simulink model "DSR_delay_beta_test"  (R2021a)
settings: Solver=VariableStepAuto  StartTime=0.0  StopTime=10  RelTol=1e-3
values from neighbouring files (symbols this model uses):
  a = 0    [gainMaxDef.m]    (also in plot2.m = 2; simulink_test.m = 5)
  alpha = 1.195    [gainMaxDef.m]    (also in plot2.m = 1.9; simulink_test.m = 1.192)
  betac = 2    [plot2.m]    (also in simulink_test.m = 10)
  c1 = 1    [simulink_test.m]
  delay = 0.5    [plot2.m]    (also in simulink_test.m = 0.015)
  delay_a = 0.150    (= 0.15)    [plot2.m]    (also in simulink_test.m = 0.01)
  gnet = 40    [plot2.m]    (also in simulink_test.m = gnetset(k))
  omega = omegalist(l)    [gainMaxDef.m]    (also in plot2.m = 300; simulink_test.m = 0.8)
  omegader = 80    [simulink_test.m]
undefined symbols (not defined in the file or in its folder): betacd
libraries: cstblocks x37, simulink x4
(part 1 of 3)
settings Model: Creator=shiva  LastModifiedBy=shiva

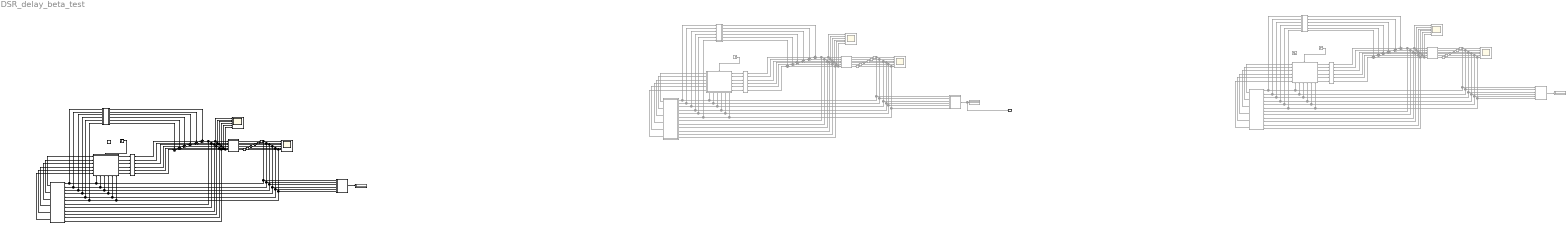
== system DSR_delay_beta_test ==
  note: DSR With CDOB
  note: DSR With CDOB
  note: DSR With CDOB
  CDOB_Subsys1 : Subsystem  Commented=on
  CDOB_Subsys2 : Subsystem  Commented=on
  CDOB_Subsys4 : Subsystem
  DSR_Input1 : Subsystem  Commented=on
      settings: PortSchema="{\"entries\":[{\"content\":{\"sides\":[{\"content\":{\"connectorIds\":[\"In1\",\"In2\",\"In3\",\"In4\",\"In5\",\"In6\"]},\"type\":\"ConnectorPlacement.EquallySpacedRectSide\",\"uuid\":\"7b8a38d4-2828-429e-a347-8750a0874c90\"},{\"content\":{\"connectorIds\":[\"Out1\",\"Out2\",\"Out3\",\"Out4\",\"Out5\",\"Out6\"],\"side\":\"RIGHT\"},\"type\":\"ConnectorPlacement.EquallySpacedRectSide\",\"uuid\":\"f1dcdaa7-0a93-43e2-be3b-ce942cee3b23\"},{\"content\":{\"connectorIds\":[\"In7\"],\"side\":\"TOP\"},\"type\":\"ConnectorPlacement.EquallySpacedRectSide\",\"uuid\":\"691a82b2-07cc-468b-b9a0-c0927a09fa47\"},{\"content\":{\"connectorIds\":[\"In8\",\"In9\",\"In10\",\"In11\",\"In12\",\"In13\"],\"side\":\"BOTTOM\"},\"type\":\"ConnectorPlacement.EquallySpacedRectSide\",\"uuid\":\"87ba8582-7e13-41cf-953e-972bab5f6463\"}]},\"type\":\"ConnectorPlacement.EquallySpacedConnector\",\"uuid\":\"6089c568-97aa-4e95-8448-5d1116d5973e\"}],\"packageUris\":[\"http://schema.mathworks.com/mf0/Connector/R2020b\"],\"version\":\"1.0\"}"
  DSR_Input2 : Subsystem  Commented=on
      settings: PortSchema="{\"entries\":[{\"content\":{\"sides\":[{\"content\":{\"connectorIds\":[\"In1\",\"In2\",\"In3\",\"In4\",\"In5\",\"In6\"]},\"type\":\"ConnectorPlacement.EquallySpacedRectSide\",\"uuid\":\"7b8a38d4-2828-429e-a347-8750a0874c90\"},{\"content\":{\"connectorIds\":[\"Out1\",\"Out2\",\"Out3\",\"Out4\",\"Out5\",\"Out6\"],\"side\":\"RIGHT\"},\"type\":\"ConnectorPlacement.EquallySpacedRectSide\",\"uuid\":\"f1dcdaa7-0a93-43e2-be3b-ce942cee3b23\"},{\"content\":{\"connectorIds\":[\"In7\"],\"side\":\"TOP\"},\"type\":\"ConnectorPlacement.EquallySpacedRectSide\",\"uuid\":\"691a82b2-07cc-468b-b9a0-c0927a09fa47\"},{\"content\":{\"connectorIds\":[\"In8\",\"In9\",\"In10\",\"In11\",\"In12\",\"In13\"],\"side\":\"BOTTOM\"},\"type\":\"ConnectorPlacement.EquallySpacedRectSide\",\"uuid\":\"87ba8582-7e13-41cf-953e-972bab5f6463\"}]},\"type\":\"ConnectorPlacement.EquallySpacedConnector\",\"uuid\":\"6089c568-97aa-4e95-8448-5d1116d5973e\"}],\"packageUris\":[\"http://schema.mathworks.com/mf0/Connector/R2020b\"],\"version\":\"1.0\"}"
  DSR_Input3 : Subsystem
      settings: PortSchema="{\"entries\":[{\"content\":{\"sides\":[{\"content\":{\"connectorIds\":[\"In1\",\"In2\",\"In3\",\"In4\",\"In5\",\"In6\"]},\"type\":\"ConnectorPlacement.EquallySpacedRectSide\",\"uuid\":\"7b8a38d4-2828-429e-a347-8750a0874c90\"},{\"content\":{\"connectorIds\":[\"Out1\",\"Out2\",\"Out3\",\"Out4\",\"Out5\",\"Out6\"],\"side\":\"RIGHT\"},\"type\":\"ConnectorPlacement.EquallySpacedRectSide\",\"uuid\":\"f1dcdaa7-0a93-43e2-be3b-ce942cee3b23\"},{\"content\":{\"connectorIds\":[\"In7\"],\"side\":\"TOP\"},\"type\":\"ConnectorPlacement.EquallySpacedRectSide\",\"uuid\":\"691a82b2-07cc-468b-b9a0-c0927a09fa47\"},{\"content\":{\"connectorIds\":[\"In8\",\"In9\",\"In10\",\"In11\",\"In12\",\"In13\"],\"side\":\"BOTTOM\"},\"type\":\"ConnectorPlacement.EquallySpacedRectSide\",\"uuid\":\"87ba8582-7e13-41cf-953e-972bab5f6463\"}]},\"type\":\"ConnectorPlacement.EquallySpacedConnector\",\"uuid\":\"6089c568-97aa-4e95-8448-5d1116d5973e\"}],\"packageUris\":[\"http://schema.mathworks.com/mf0/Connector/R2020b\"],\"version\":\"1.0\"}"
  Display1 : Display  Commented=on
  Display2 : Display
  Display3 : Display  Commented=on
  Max Deflection1 : Subsystem  Commented=on
  Max Deflection2 : Subsystem  Commented=on
  Max Deflection3 : Subsystem
  Ramp : simulink/Sources/Ramp  slope=1  start=0  InitialOutput=0
  Scope{1..4} (4 alike) : Scope  Commented=on  NumInputPorts=6
  Scope5 : Scope  NumInputPorts=6
  Scope6 : Scope  NumInputPorts=6
  Sine Wave1 : Sin  Commented=on  SampleTime=0
  StateDerivative1 : Subsystem  Commented=on
  StateDerivative2 : Subsystem  Commented=on
  StateDerivative3 : Subsystem
  Step1 : Step  Commented=on  Time=0  SampleTime=0
  Step2 : Step  Commented=on  Time=0  SampleTime=0
  Step3 : Step  Time=0  SampleTime=0
  Subsystem1 : Subsystem  Commented=on
  Subsystem2 : Subsystem
  Subsystem3 : Subsystem  Commented=on
  Sum{1..12} (12 alike) : Sum  Commented=on  Inputs=++|
  Sum{13..18} (6 alike) : Sum  Inputs=++|
  Transport Delay{1..12} (12 alike) : TransportDelay  Commented=on  DelayTime=delay_a
  Transport Delay{13..18} (6 alike) : TransportDelay  DelayTime=delay_a
  gain 1/a1 : Subsystem  Commented=on
  gain 1/a2 : Subsystem  Commented=on
  gain 1/a3 : Subsystem
  Output : Outport
  wires:
  Max Deflection1/1(y) -> Output/1, Display3/1
  Transport Delay3/1 -> StateDerivative1/2(Input1), CDOB_Subsys2/2(XRes1), DSR_Input1/9(s2), Max Deflection1/2(In2), Scope1/2
  Sum2/1 -> CDOB_Subsys2/8(Acc.1), Subsystem3/2(In2), Scope2/2
  DSR_Input1/1(Out1) -> gain 1/a1/1(In1)
  gain 1/a1/5(Out5) -> Sum5/2
  CDOB_Subsys2/4(FeedBack3) -> DSR_Input1/4(fb4)
  DSR_Input1/2(Out2) -> gain 1/a1/2(In2)
  Subsystem3/5(O5) -> Transport Delay11/1
  Subsystem3/2(O2) -> Transport Delay3/1
  DSR_Input1/4(Out4) -> gain 1/a1/4(In4)
  CDOB_Subsys2/1(FeedBack) -> DSR_Input1/1(fb1)
  gain 1/a1/6(Out6) -> Sum6/2
  Subsystem3/6(O6) -> Transport Delay2/1
  Sum4/1 -> CDOB_Subsys2/10(Acc.3), Scope2/4, Subsystem3/4(In4)
  DSR_Input1/6(Out6) -> gain 1/a1/6(In6)
  Transport Delay11/1 -> StateDerivative1/5(Input4), CDOB_Subsys2/5(XRes4), DSR_Input1/12(s5), Max Deflection1/5(In5), Scope1/5
  gain 1/a1/1(Out1) -> Sum1/2
  gain 1/a1/3(Out3) -> Sum3/2
  Sum6/1 -> Scope2/6, Subsystem3/6(In6), CDOB_Subsys2/12(Acc.5)
  DSR_Input1/5(Out5) -> gain 1/a1/5(In5)
  Subsystem3/3(O3) -> Transport Delay4/1
  DSR_Input1/3(Out3) -> gain 1/a1/3(In3)
  Sum3/1 -> CDOB_Subsys2/9(Acc.2), Scope2/3, Subsystem3/3(In3)
  Subsystem3/4(O4) -> Transport Delay5/1
  Transport Delay1/1 -> Scope1/1, StateDerivative1/1(Input), CDOB_Subsys2/1(XRes), DSR_Input1/8(s1), Max Deflection1/1(In1)
  Sum1/1 -> CDOB_Subsys2/7(Acc.), Subsystem3/1(In1), Scope2/1
  CDOB_Subsys2/5(FeedBack4) -> DSR_Input1/5(fb5)
  CDOB_Subsys2/6(FeedBack5) -> DSR_Input1/6(fb6)
  gain 1/a1/4(Out4) -> Sum4/2
  Transport Delay2/1 -> Scope1/6, StateDerivative1/6(Input5), CDOB_Subsys2/6(XRes5), DSR_Input1/13(s6), Max Deflection1/6(In6)
  gain 1/a1/2(Out2) -> Sum2/2
  Subsystem3/1(O1) -> Transport Delay1/1
  Transport Delay5/1 -> StateDerivative1/4(Input3), CDOB_Subsys2/4(XRes3), DSR_Input1/11(s4), Max Deflection1/4(In4), Scope1/4
  Transport Delay4/1 -> StateDerivative1/3(Input2), CDOB_Subsys2/3(XRes2), DSR_Input1/10(s3), Max Deflection1/3(In3), Scope1/3
  CDOB_Subsys2/2(FeedBack1) -> DSR_Input1/2(fb2)
  CDOB_Subsys2/3(FeedBack2) -> DSR_Input1/3(fb3)
  Sum5/1 -> CDOB_Subsys2/11(Acc.4), Scope2/5, Subsystem3/5(In5)
  StateDerivative1/1(Out1) -> Sum1/1
  StateDerivative1/2(Out2) -> Sum2/1
  StateDerivative1/3(Out3) -> Sum3/1
  StateDerivative1/4(Out4) -> Sum4/1
  StateDerivative1/5(Out5) -> Sum5/1
  StateDerivative1/6(Out6) -> Sum6/1
  Step1/1 -> DSR_Input1/7(input)
  StateDerivative2/4(Out4) -> Sum10/1
  StateDerivative2/2(Out2) -> Sum8/1
  StateDerivative2/3(Out3) -> Sum9/1
  StateDerivative2/1(Out1) -> Sum7/1
  Step2/1 -> DSR_Input2/7(input)
  DSR_Input2/2(Out2) -> gain 1/a2/2(In2)
  Max Deflection2/1(y) -> Display1/1
  Transport Delay10/1 -> StateDerivative2/3(Input2), CDOB_Subsys1/3(XRes2), DSR_Input2/10(s3), Max Deflection2/3(In3), Scope3/3
  Transport Delay12/1 -> StateDerivative2/4(Input3), CDOB_Subsys1/4(XRes3), DSR_Input2/11(s4), Max Deflection2/4(In4), Scope3/4
  Sum11/1 -> CDOB_Subsys1/11(Acc.4), Scope4/5, Subsystem1/5(In5)
  CDOB_Subsys1/3(FeedBack2) -> DSR_Input2/3(fb3)
  CDOB_Subsys1/2(FeedBack1) -> DSR_Input2/2(fb2)
  gain 1/a2/4(Out4) -> Sum10/2
  CDOB_Subsys1/6(FeedBack5) -> DSR_Input2/6(fb6)
  Subsystem1/4(O4) -> Transport Delay12/1
  CDOB_Subsys1/5(FeedBack4) -> DSR_Input2/5(fb5)
  Sum9/1 -> CDOB_Subsys1/9(Acc.2), Scope4/3, Subsystem1/3(In3)
  DSR_Input2/3(Out3) -> gain 1/a2/3(In3)
  StateDerivative2/6(Out6) -> Sum12/1
  Sum12/1 -> Scope4/6, Subsystem1/6(In6), CDOB_Subsys1/12(Acc.5)
  DSR_Input2/5(Out5) -> gain 1/a2/5(In5)
  gain 1/a2/1(Out1) -> Sum7/2
  Transport Delay7/1 -> StateDerivative2/5(Input4), CDOB_Subsys1/5(XRes4), DSR_Input2/12(s5), Max Deflection2/5(In5), Scope3/5
  gain 1/a2/3(Out3) -> Sum9/2
  gain 1/a2/2(Out2) -> Sum8/2
  Subsystem1/2(O2) -> Transport Delay9/1
  Subsystem1/6(O6) -> Transport Delay8/1
  Subsystem1/3(O3) -> Transport Delay10/1
  gain 1/a2/6(Out6) -> Sum12/2
  Sum10/1 -> CDOB_Subsys1/10(Acc.3), Scope4/4, Subsystem1/4(In4)
  Sum7/1 -> CDOB_Subsys1/7(Acc.), Subsystem1/1(In1), Scope4/1
  CDOB_Subsys1/1(FeedBack) -> DSR_Input2/1(fb1)
  DSR_Input2/4(Out4) -> gain 1/a2/4(In4)
  Subsystem1/5(O5) -> Transport Delay7/1
  Sum8/1 -> CDOB_Subsys1/8(Acc.1), Subsystem1/2(In2), Scope4/2
  CDOB_Subsys1/4(FeedBack3) -> DSR_Input2/4(fb4)
  DSR_Input2/6(Out6) -> gain 1/a2/6(In6)
  Transport Delay6/1 -> Scope3/1, StateDerivative2/1(Input), CDOB_Subsys1/1(XRes), DSR_Input2/8(s1), Max Deflection2/1(In1)
  StateDerivative2/5(Out5) -> Sum11/1
  Transport Delay8/1 -> StateDerivative2/6(Input5), CDOB_Subsys1/6(XRes5), DSR_Input2/13(s6), Max Deflection2/6(In6), Scope3/6
  gain 1/a2/5(Out5) -> Sum11/2
  DSR_Input2/1(Out1) -> gain 1/a2/1(In1)
  Subsystem1/1(O1) -> Transport Delay6/1
  Transport Delay9/1 -> StateDerivative2/2(Input1), CDOB_Subsys1/2(XRes1), DSR_Input2/9(s2), Max Deflection2/2(In2), Scope3/2
  StateDerivative3/3(Out3) -> Sum15/1
  DSR_Input3/6(Out6) -> gain 1/a3/6(In6)
  Transport Delay18/1 -> CDOB_Subsys4/4(XRes3), StateDerivative3/4(Input3), DSR_Input3/11(s4), Max Deflection3/4(In4), Scope5/4
  Sum13/1 -> CDOB_Subsys4/7(Acc.), Subsystem2/1(In1), Scope6/1
  gain 1/a3/2(Out2) -> Sum14/2
  gain 1/a3/3(Out3) -> Sum15/2
  StateDerivative3/2(Out2) -> Sum14/1
  gain 1/a3/5(Out5) -> Sum17/2
  CDOB_Subsys4/3(FeedBack2) -> DSR_Input3/3(fb3)
  Transport Delay16/1 -> CDOB_Subsys4/2(XRes1), StateDerivative3/2(Input1), DSR_Input3/9(s2), Max Deflection3/2(In2), Scope5/2
  DSR_Input3/3(Out3) -> gain 1/a3/3(In3)
  DSR_Input3/1(Out1) -> gain 1/a3/1(In1)
  Transport Delay17/1 -> CDOB_Subsys4/3(XRes2), StateDerivative3/3(Input2), DSR_Input3/10(s3), Max Deflection3/3(In3), Scope5/3
  Transport Delay14/1 -> CDOB_Subsys4/5(XRes4), StateDerivative3/5(Input4), DSR_Input3/12(s5), Max Deflection3/5(In5), Scope5/5
  Subsystem2/1(O1) -> Transport Delay13/1
  Transport Delay13/1 -> Scope5/1, CDOB_Subsys4/1(XRes), StateDerivative3/1(Input), DSR_Input3/8(s1), Max Deflection3/1(In1)
  StateDerivative3/4(Out4) -> Sum16/1
  StateDerivative3/1(Out1) -> Sum13/1
  gain 1/a3/4(Out4) -> Sum16/2
  CDOB_Subsys4/5(FeedBack4) -> DSR_Input3/5(fb5)
  Transport Delay15/1 -> Scope5/6, CDOB_Subsys4/6(XRes5), StateDerivative3/6(Input5), DSR_Input3/13(s6), Max Deflection3/6(In6)
  CDOB_Subsys4/1(FeedBack) -> DSR_Input3/1(fb1)
  Subsystem2/4(O4) -> Transport Delay18/1
  Sum17/1 -> CDOB_Subsys4/11(Acc.4), Scope6/5, Subsystem2/5(In5)
  CDOB_Subsys4/6(FeedBack5) -> DSR_Input3/6(fb6)
  Sum15/1 -> CDOB_Subsys4/9(Acc.2), Scope6/3, Subsystem2/3(In3)
  DSR_Input3/4(Out4) -> gain 1/a3/4(In4)
  Subsystem2/3(O3) -> Transport Delay17/1
  Subsystem2/2(O2) -> Transport Delay16/1
  Sum18/1 -> CDOB_Subsys4/12(Acc.5), Scope6/6, Subsystem2/6(In6)
  CDOB_Subsys4/4(FeedBack3) -> DSR_Input3/4(fb4)
  DSR_Input3/2(Out2) -> gain 1/a3/2(In2)
  Subsystem2/6(O6) -> Transport Delay15/1
  gain 1/a3/1(Out1) -> Sum13/2
  Sum16/1 -> CDOB_Subsys4/10(Acc.3), Scope6/4, Subsystem2/4(In4)
  gain 1/a3/6(Out6) -> Sum18/2
  DSR_Input3/5(Out5) -> gain 1/a3/5(In5)
  Max Deflection3/1(y) -> Display2/1
  StateDerivative3/5(Out5) -> Sum17/1
  StateDerivative3/6(Out6) -> Sum18/1
  Subsystem2/5(O5) -> Transport Delay14/1
  Sum14/1 -> CDOB_Subsys4/8(Acc.1), Subsystem2/2(In2), Scope6/2
  CDOB_Subsys4/2(FeedBack1) -> DSR_Input3/2(fb2)
  Step3/1 -> DSR_Input3/7(input)

== system DSR_delay_beta_test/CDOB_Subsys1 ==
  XRes : Inport
  XRes1 : Inport  Port=2
  XRes2 : Inport  Port=3
  XRes3 : Inport  Port=4
  XRes4 : Inport  Port=5
  XRes5 : Inport  Port=6
  Acc. : Inport  Port=7
  Acc.1 : Inport  Port=8
  Acc.2 : Inport  Port=9
  Acc.3 : Inport  Port=10
  Acc.4 : Inport  Port=11
  Acc.5 : Inport  Port=12
  ND : Subsystem
  ND1 : Subsystem
  ND2 : Subsystem
  ND3 : Subsystem
  ND4 : Subsystem
  ND5 : Subsystem
  FeedBack : Outport
  FeedBack1 : Outport  Port=2
  FeedBack2 : Outport  Port=3
  FeedBack3 : Outport  Port=4
  FeedBack4 : Outport  Port=5
  FeedBack5 : Outport  Port=6
  wires:
  Acc./1 -> ND/2(Acc.)
  XRes/1 -> ND/1(XRes)
  Acc.4/1 -> ND4/2(Acc.)
  Acc.3/1 -> ND3/2(Acc.)
  XRes1/1 -> ND1/1(XRes)
  XRes2/1 -> ND2/1(XRes)
  XRes4/1 -> ND4/1(XRes)
  XRes5/1 -> ND5/1(XRes)
  Acc.2/1 -> ND2/2(Acc.)
  ND5/1(FeedBack) -> FeedBack5/1
  ND1/1(FeedBack) -> FeedBack1/1
  ND2/1(FeedBack) -> FeedBack2/1
  Acc.5/1 -> ND5/2(Acc.)
  ND4/1(FeedBack) -> FeedBack4/1
  ND/1(FeedBack) -> FeedBack/1
  ND3/1(FeedBack) -> FeedBack3/1
  XRes3/1 -> ND3/1(XRes)
  Acc.1/1 -> ND1/2(Acc.)

== system DSR_delay_beta_test/CDOB_Subsys2 ==
  XRes : Inport
  XRes1 : Inport  Port=2
  XRes2 : Inport  Port=3
  XRes3 : Inport  Port=4
  XRes4 : Inport  Port=5
  XRes5 : Inport  Port=6
  Acc. : Inport  Port=7
  Acc.1 : Inport  Port=8
  Acc.2 : Inport  Port=9
  Acc.3 : Inport  Port=10
  Acc.4 : Inport  Port=11
  Acc.5 : Inport  Port=12
  ND : Subsystem
  ND1 : Subsystem
  ND2 : Subsystem
  ND3 : Subsystem
  ND4 : Subsystem
  ND5 : Subsystem
  FeedBack : Outport
  FeedBack1 : Outport  Port=2
  FeedBack2 : Outport  Port=3
  FeedBack3 : Outport  Port=4
  FeedBack4 : Outport  Port=5
  FeedBack5 : Outport  Port=6
  wires:
  Acc./1 -> ND/2(Acc.)
  XRes/1 -> ND/1(XRes)
  Acc.4/1 -> ND4/2(Acc.)
  Acc.3/1 -> ND3/2(Acc.)
  XRes1/1 -> ND1/1(XRes)
  XRes2/1 -> ND2/1(XRes)
  XRes4/1 -> ND4/1(XRes)
  XRes5/1 -> ND5/1(XRes)
  Acc.2/1 -> ND2/2(Acc.)
  ND5/1(FeedBack) -> FeedBack5/1
  ND1/1(FeedBack) -> FeedBack1/1
  ND2/1(FeedBack) -> FeedBack2/1
  Acc.5/1 -> ND5/2(Acc.)
  ND4/1(FeedBack) -> FeedBack4/1
  ND/1(FeedBack) -> FeedBack/1
  ND3/1(FeedBack) -> FeedBack3/1
  XRes3/1 -> ND3/1(XRes)
  Acc.1/1 -> ND1/2(Acc.)

== system DSR_delay_beta_test/CDOB_Subsys4 ==
  XRes : Inport
  XRes1 : Inport  Port=2
  XRes2 : Inport  Port=3
  XRes3 : Inport  Port=4
  XRes4 : Inport  Port=5
  XRes5 : Inport  Port=6
  Acc. : Inport  Port=7
  Acc.1 : Inport  Port=8
  Acc.2 : Inport  Port=9
  Acc.3 : Inport  Port=10
  Acc.4 : Inport  Port=11
  Acc.5 : Inport  Port=12
  ND : Subsystem
  ND1 : Subsystem
  ND2 : Subsystem
  ND3 : Subsystem
  ND4 : Subsystem
  ND5 : Subsystem
  FeedBack : Outport
  FeedBack1 : Outport  Port=2
  FeedBack2 : Outport  Port=3
  FeedBack3 : Outport  Port=4
  FeedBack4 : Outport  Port=5
  FeedBack5 : Outport  Port=6
  wires:
  Acc./1 -> ND/2(Acc.)
  XRes/1 -> ND/1(XRes)
  Acc.4/1 -> ND4/2(Acc.)
  Acc.3/1 -> ND3/2(Acc.)
  XRes1/1 -> ND1/1(XRes)
  XRes2/1 -> ND2/1(XRes)
  XRes4/1 -> ND4/1(XRes)
  XRes5/1 -> ND5/1(XRes)
  Acc.2/1 -> ND2/2(Acc.)
  ND5/1(FeedBack) -> FeedBack5/1
  ND1/1(FeedBack) -> FeedBack1/1
  ND2/1(FeedBack) -> FeedBack2/1
  Acc.5/1 -> ND5/2(Acc.)
  ND4/1(FeedBack) -> FeedBack4/1
  ND/1(FeedBack) -> FeedBack/1
  ND3/1(FeedBack) -> FeedBack3/1
  XRes3/1 -> ND3/1(XRes)
  Acc.1/1 -> ND1/2(Acc.)

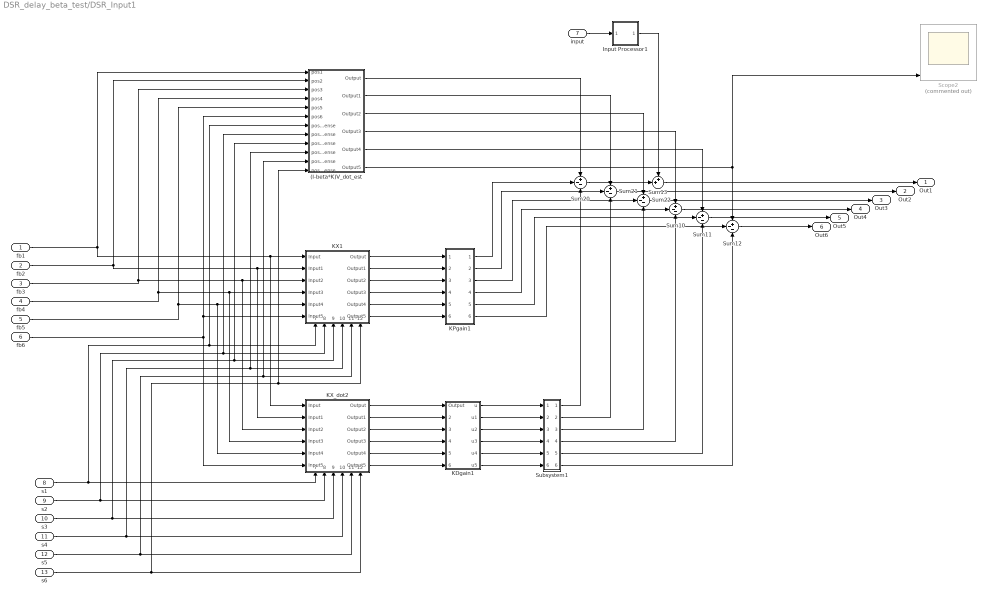
== system DSR_delay_beta_test/DSR_Input1 ==
  fb1 : Inport
  fb2 : Inport  Port=2
  fb3 : Inport  Port=3
  fb4 : Inport  Port=4
  fb5 : Inport  Port=5
  fb6 : Inport  Port=6
  input : Inport  Port=7
  s1 : Inport  Port=8
  s2 : Inport  Port=9
  s3 : Inport  Port=10
  s4 : Inport  Port=11
  s5 : Inport  Port=12
  s6 : Inport  Port=13
  (I-beta*K)V_dot_est : Subsystem
  Input Processor1 : Subsystem
  KDgain1 : Subsystem
  KPgain1 : Subsystem
  KX1 : Subsystem
      settings: PortSchema="{\"entries\":[{\"content\":{\"sides\":[{\"content\":{\"connectorIds\":[\"In1\",\"In2\",\"In3\",\"In4\",\"In5\",\"In6\"]},\"type\":\"ConnectorPlacement.EquallySpacedRectSide\",\"uuid\":\"24ff0189-2e26-4de2-9c90-2043606e3d63\"},{\"content\":{\"connectorIds\":[\"Out1\",\"Out2\",\"Out3\",\"Out4\",\"Out5\",\"Out6\"],\"side\":\"RIGHT\"},\"type\":\"ConnectorPlacement.EquallySpacedRectSide\",\"uuid\":\"7efe01dd-8101-429e-adc6-a10b45356e48\"},{\"content\":{\"connectorIds\":[],\"side\":\"TOP\"},\"type\":\"ConnectorPlacement.EquallySpacedRectSide\",\"uuid\":\"5c1fc1f4-b8b0-4afd-80fe-11f4d157d0fc\"},{\"content\":{\"connectorIds\":[\"In7\",\"In8\",\"In9\",\"In10\",\"In11\",\"In12\"],\"side\":\"BOTTOM\"},\"type\":\"ConnectorPlacement.EquallySpacedRectSide\",\"uuid\":\"e52c51d8-b236-4cc8-9958-a8d91e3741c4\"}]},\"type\":\"ConnectorPlacement.EquallySpacedConnector\",\"uuid\":\"3e3502e3-b8a3-4e9d-9b78-ab08dd870d4b\"}],\"packageUris\":[\"http://schema.mathworks.com/mf0/Connector/R2020b\"],\"version\":\"1.0\"}"
  KX_dot2 : Subsystem
      settings: PortSchema="{\"entries\":[{\"content\":{\"sides\":[{\"content\":{\"connectorIds\":[\"In1\",\"In2\",\"In3\",\"In4\",\"In5\",\"In6\"]},\"type\":\"ConnectorPlacement.EquallySpacedRectSide\",\"uuid\":\"24ff0189-2e26-4de2-9c90-2043606e3d63\"},{\"content\":{\"connectorIds\":[\"Out1\",\"Out2\",\"Out3\",\"Out4\",\"Out5\",\"Out6\"],\"side\":\"RIGHT\"},\"type\":\"ConnectorPlacement.EquallySpacedRectSide\",\"uuid\":\"7efe01dd-8101-429e-adc6-a10b45356e48\"},{\"content\":{\"connectorIds\":[],\"side\":\"TOP\"},\"type\":\"ConnectorPlacement.EquallySpacedRectSide\",\"uuid\":\"5c1fc1f4-b8b0-4afd-80fe-11f4d157d0fc\"},{\"content\":{\"connectorIds\":[\"In7\",\"In8\",\"In9\",\"In10\",\"In11\",\"In12\"],\"side\":\"BOTTOM\"},\"type\":\"ConnectorPlacement.EquallySpacedRectSide\",\"uuid\":\"bae418dc-ca78-4370-85bb-31cb43009c14\"}]},\"type\":\"ConnectorPlacement.EquallySpacedConnector\",\"uuid\":\"3e3502e3-b8a3-4e9d-9b78-ab08dd870d4b\"}],\"packageUris\":[\"http://schema.mathworks.com/mf0/Connector/R2020b\"],\"version\":\"1.0\"}"
  Scope2 : Scope  Commented=on  NumInputPorts=6
  Subsystem1 : Subsystem
  Sum{10..12,20..22} (6 alike) : Sum  Inputs=+--
  Sum13 : Sum  Inputs=++|
  Out1 : Outport
  Out2 : Outport  Port=2
  Out3 : Outport  Port=3
  Out4 : Outport  Port=4
  Out5 : Outport  Port=5
  Out6 : Outport  Port=6
  wires:
  KX_dot2/5(Output4) -> KDgain1/5(Output4)
  fb4/1 -> KX1/4(Input3), KX_dot2/4(Input3), (I-beta*K)V_dot_est/4(pos4)
  fb2/1 -> KX1/2(Input1), KX_dot2/2(Input1), (I-beta*K)V_dot_est/2(pos2)
  KDgain1/6(u5) -> Subsystem1/6(u5)
  fb3/1 -> KX1/3(Input2), KX_dot2/3(Input2), (I-beta*K)V_dot_est/3(pos3)
  KPgain1/4(Out4) -> Sum10/2
  Sum10/1 -> Out4/1
  KPgain1/2(Out2) -> Sum21/2
  KX1/6(Output5) -> KPgain1/6(Output5)
  KX1/2(Output1) -> KPgain1/2(Output1)
  KPgain1/6(Out6) -> Sum12/2
  KX1/4(Output3) -> KPgain1/4(Output3)
  KX1/3(Output2) -> KPgain1/3(Output2)
  s6/1 -> KX_dot2/12(sense6), (I-beta*K)V_dot_est/12(pos6sense), KX1/12(sense6)
  KDgain1/4(u3) -> Subsystem1/4(u3)
  fb5/1 -> KX1/5(Input4), KX_dot2/5(Input4), (I-beta*K)V_dot_est/5(pos5)
  Sum22/1 -> Out3/1
  Sum12/1 -> Out6/1
  KPgain1/3(Out3) -> Sum22/2
  KDgain1/5(u4) -> Subsystem1/5(u4)
  KDgain1/2(u1) -> Subsystem1/2(u1)
  s3/1 -> KX_dot2/9(sense3), (I-beta*K)V_dot_est/9(pos3sense), KX1/9(sense3)
  Sum20/1 -> Sum13/2
  KDgain1/3(u2) -> Subsystem1/3(u2)
  KX_dot2/4(Output3) -> KDgain1/4(Output3)
  fb1/1 -> KX1/1(Input), KX_dot2/1(Input), (I-beta*K)V_dot_est/1(pos1)
  (I-beta*K)V_dot_est/1(Output) -> Sum20/1
  KX_dot2/6(Output5) -> KDgain1/6(Output5)
  s1/1 -> KX_dot2/7(sense1), (I-beta*K)V_dot_est/7(pos1sense), KX1/7(sense1)
  s5/1 -> KX_dot2/11(sense5), (I-beta*K)V_dot_est/11(pos5sense), KX1/11(sense5)
  KX_dot2/2(Output1) -> KDgain1/2(Output1)
  Sum21/1 -> Out2/1
  KPgain1/5(Out5) -> Sum11/2
  fb6/1 -> KX1/6(Input5), (I-beta*K)V_dot_est/6(pos6), KX_dot2/6(Input5)
  (I-beta*K)V_dot_est/3(Output2) -> Sum22/1
  s4/1 -> KX_dot2/10(sense4), (I-beta*K)V_dot_est/10(pos4sense), KX1/10(sense4)
  KX1/5(Output4) -> KPgain1/5(Output4)
  KDgain1/1(u) -> Subsystem1/1(u)
  KX1/1(Output) -> KPgain1/1(Output)
  input/1 -> Input Processor1/1(Input)
  (I-beta*K)V_dot_est/2(Output1) -> Sum21/1
  KX_dot2/3(Output2) -> KDgain1/3(Output2)
  Sum11/1 -> Out5/1
  (I-beta*K)V_dot_est/4(Output3) -> Sum10/1
  KX_dot2/1(Output) -> KDgain1/1(Output)
  (I-beta*K)V_dot_est/5(Output4) -> Sum11/1
  (I-beta*K)V_dot_est/6(Output5) -> Scope2/6, Sum12/1
  KPgain1/1(Out1) -> Sum20/2
  s2/1 -> KX_dot2/8(sense2), (I-beta*K)V_dot_est/8(pos2sense), KX1/8(sense2)
  Sum13/1 -> Out1/1
  Input Processor1/1(Out1) -> Sum13/1
  Subsystem1/1(Out7) -> Sum20/3
  Subsystem1/2(Out8) -> Sum21/3
  Subsystem1/3(Out9) -> Sum22/3
  Subsystem1/4(Out10) -> Sum10/3
  Subsystem1/5(Out11) -> Sum11/3
  Subsystem1/6(Out12) -> Sum12/3

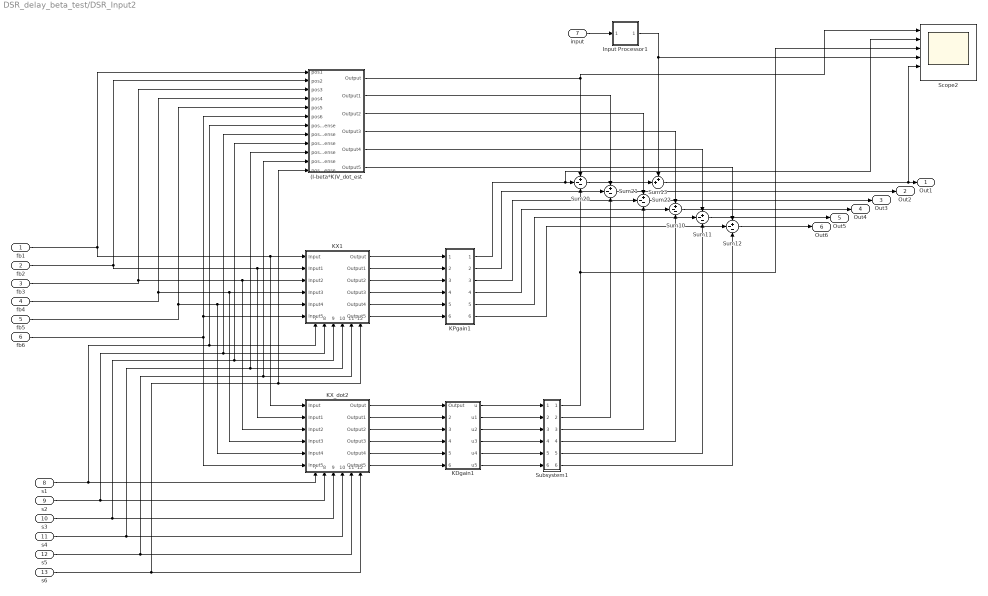
== system DSR_delay_beta_test/DSR_Input2 ==
  fb1 : Inport
  fb2 : Inport  Port=2
  fb3 : Inport  Port=3
  fb4 : Inport  Port=4
  fb5 : Inport  Port=5
  fb6 : Inport  Port=6
  input : Inport  Port=7
  s1 : Inport  Port=8
  s2 : Inport  Port=9
  s3 : Inport  Port=10
  s4 : Inport  Port=11
  s5 : Inport  Port=12
  s6 : Inport  Port=13
  (I-beta*K)V_dot_est : Subsystem
  Input Processor1 : Subsystem
  KDgain1 : Subsystem
  KPgain1 : Subsystem
  KX1 : Subsystem
      settings: PortSchema="{\"entries\":[{\"content\":{\"sides\":[{\"content\":{\"connectorIds\":[\"In1\",\"In2\",\"In3\",\"In4\",\"In5\",\"In6\"]},\"type\":\"ConnectorPlacement.EquallySpacedRectSide\",\"uuid\":\"24ff0189-2e26-4de2-9c90-2043606e3d63\"},{\"content\":{\"connectorIds\":[\"Out1\",\"Out2\",\"Out3\",\"Out4\",\"Out5\",\"Out6\"],\"side\":\"RIGHT\"},\"type\":\"ConnectorPlacement.EquallySpacedRectSide\",\"uuid\":\"7efe01dd-8101-429e-adc6-a10b45356e48\"},{\"content\":{\"connectorIds\":[],\"side\":\"TOP\"},\"type\":\"ConnectorPlacement.EquallySpacedRectSide\",\"uuid\":\"5c1fc1f4-b8b0-4afd-80fe-11f4d157d0fc\"},{\"content\":{\"connectorIds\":[\"In7\",\"In8\",\"In9\",\"In10\",\"In11\",\"In12\"],\"side\":\"BOTTOM\"},\"type\":\"ConnectorPlacement.EquallySpacedRectSide\",\"uuid\":\"e52c51d8-b236-4cc8-9958-a8d91e3741c4\"}]},\"type\":\"ConnectorPlacement.EquallySpacedConnector\",\"uuid\":\"3e3502e3-b8a3-4e9d-9b78-ab08dd870d4b\"}],\"packageUris\":[\"http://schema.mathworks.com/mf0/Connector/R2020b\"],\"version\":\"1.0\"}"
  KX_dot2 : Subsystem
      settings: PortSchema="{\"entries\":[{\"content\":{\"sides\":[{\"content\":{\"connectorIds\":[\"In1\",\"In2\",\"In3\",\"In4\",\"In5\",\"In6\"]},\"type\":\"ConnectorPlacement.EquallySpacedRectSide\",\"uuid\":\"24ff0189-2e26-4de2-9c90-2043606e3d63\"},{\"content\":{\"connectorIds\":[\"Out1\",\"Out2\",\"Out3\",\"Out4\",\"Out5\",\"Out6\"],\"side\":\"RIGHT\"},\"type\":\"ConnectorPlacement.EquallySpacedRectSide\",\"uuid\":\"7efe01dd-8101-429e-adc6-a10b45356e48\"},{\"content\":{\"connectorIds\":[],\"side\":\"TOP\"},\"type\":\"ConnectorPlacement.EquallySpacedRectSide\",\"uuid\":\"5c1fc1f4-b8b0-4afd-80fe-11f4d157d0fc\"},{\"content\":{\"connectorIds\":[\"In7\",\"In8\",\"In9\",\"In10\",\"In11\",\"In12\"],\"side\":\"BOTTOM\"},\"type\":\"ConnectorPlacement.EquallySpacedRectSide\",\"uuid\":\"bae418dc-ca78-4370-85bb-31cb43009c14\"}]},\"type\":\"ConnectorPlacement.EquallySpacedConnector\",\"uuid\":\"3e3502e3-b8a3-4e9d-9b78-ab08dd870d4b\"}],\"packageUris\":[\"http://schema.mathworks.com/mf0/Connector/R2020b\"],\"version\":\"1.0\"}"
  Scope2 : Scope  NumInputPorts=6
  Subsystem1 : Subsystem
  Sum{10..12,20..22} (6 alike) : Sum  Inputs=+--
  Sum13 : Sum  Inputs=++|
  Out1 : Outport
  Out2 : Outport  Port=2
  Out3 : Outport  Port=3
  Out4 : Outport  Port=4
  Out5 : Outport  Port=5
  Out6 : Outport  Port=6
  wires:
  KX_dot2/5(Output4) -> KDgain1/5(Output4)
  fb4/1 -> KX1/4(Input3), KX_dot2/4(Input3), (I-beta*K)V_dot_est/4(pos4)
  fb2/1 -> KX1/2(Input1), KX_dot2/2(Input1), (I-beta*K)V_dot_est/2(pos2)
  KDgain1/6(u5) -> Subsystem1/6(u5)
  fb3/1 -> KX1/3(Input2), KX_dot2/3(Input2), (I-beta*K)V_dot_est/3(pos3)
  KPgain1/4(Out4) -> Sum10/2
  Sum10/1 -> Out4/1
  KPgain1/2(Out2) -> Sum21/2
  KX1/6(Output5) -> KPgain1/6(Output5)
  KX1/2(Output1) -> KPgain1/2(Output1)
  KPgain1/6(Out6) -> Sum12/2
  KX1/4(Output3) -> KPgain1/4(Output3)
  KX1/3(Output2) -> KPgain1/3(Output2)
  s6/1 -> KX_dot2/12(sense6), (I-beta*K)V_dot_est/12(pos6sense), KX1/12(sense6)
  KDgain1/4(u3) -> Subsystem1/4(u3)
  fb5/1 -> KX1/5(Input4), KX_dot2/5(Input4), (I-beta*K)V_dot_est/5(pos5)
  Sum22/1 -> Out3/1
  Sum12/1 -> Out6/1
  KPgain1/3(Out3) -> Sum22/2
  KDgain1/5(u4) -> Subsystem1/5(u4)
  KDgain1/2(u1) -> Subsystem1/2(u1)
  s3/1 -> KX_dot2/9(sense3), (I-beta*K)V_dot_est/9(pos3sense), KX1/9(sense3)
  Sum20/1 -> Sum13/2
  KDgain1/3(u2) -> Subsystem1/3(u2)
  KX_dot2/4(Output3) -> KDgain1/4(Output3)
  fb1/1 -> KX1/1(Input), KX_dot2/1(Input), (I-beta*K)V_dot_est/1(pos1)
  (I-beta*K)V_dot_est/1(Output) -> Scope2/1, Sum20/1
  KX_dot2/6(Output5) -> KDgain1/6(Output5)
  s1/1 -> KX_dot2/7(sense1), (I-beta*K)V_dot_est/7(pos1sense), KX1/7(sense1)
  s5/1 -> KX_dot2/11(sense5), (I-beta*K)V_dot_est/11(pos5sense), KX1/11(sense5)
  KX_dot2/2(Output1) -> KDgain1/2(Output1)
  Sum21/1 -> Out2/1
  KPgain1/5(Out5) -> Sum11/2
  fb6/1 -> KX1/6(Input5), (I-beta*K)V_dot_est/6(pos6), KX_dot2/6(Input5)
  (I-beta*K)V_dot_est/3(Output2) -> Sum22/1
  s4/1 -> KX_dot2/10(sense4), (I-beta*K)V_dot_est/10(pos4sense), KX1/10(sense4)
  KX1/5(Output4) -> KPgain1/5(Output4)
  KDgain1/1(u) -> Subsystem1/1(u)
  KX1/1(Output) -> KPgain1/1(Output)
  input/1 -> Input Processor1/1(Input)
  (I-beta*K)V_dot_est/2(Output1) -> Sum21/1
  KX_dot2/3(Output2) -> KDgain1/3(Output2)
  Sum11/1 -> Out5/1
  (I-beta*K)V_dot_est/4(Output3) -> Sum10/1
  KX_dot2/1(Output) -> KDgain1/1(Output)
  (I-beta*K)V_dot_est/5(Output4) -> Sum11/1
  (I-beta*K)V_dot_est/6(Output5) -> Sum12/1
  KPgain1/1(Out1) -> Scope2/2, Sum20/2
  s2/1 -> KX_dot2/8(sense2), (I-beta*K)V_dot_est/8(pos2sense), KX1/8(sense2)
  Sum13/1 -> Scope2/5, Out1/1
  Input Processor1/1(Out1) -> Scope2/4, Sum13/1
  Subsystem1/1(Out7) -> Scope2/3, Sum20/3
  Subsystem1/2(Out8) -> Sum21/3
  Subsystem1/3(Out9) -> Sum22/3
  Subsystem1/4(Out10) -> Sum10/3
  Subsystem1/5(Out11) -> Sum11/3
  Subsystem1/6(Out12) -> Sum12/3

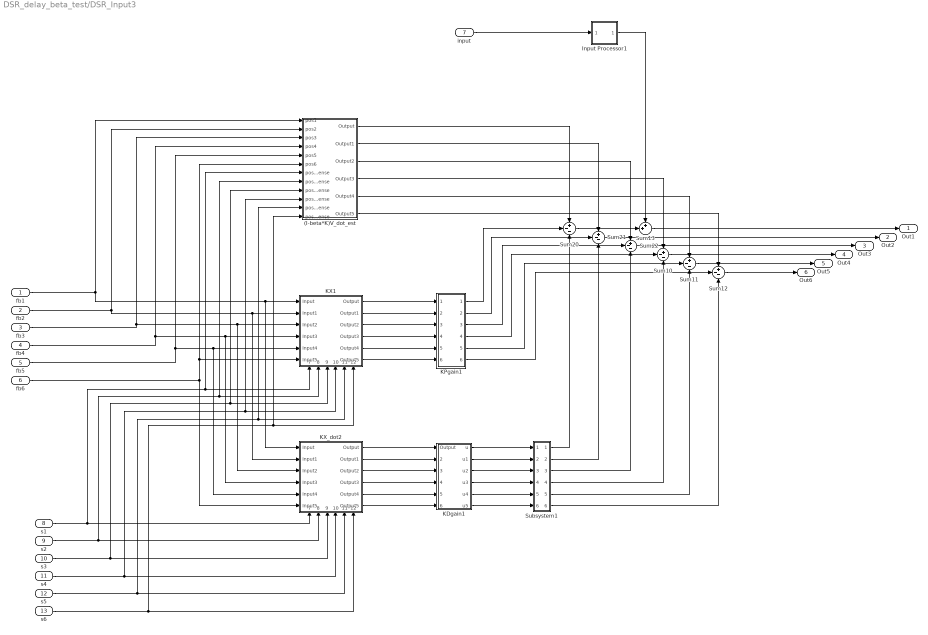
== system DSR_delay_beta_test/DSR_Input3 ==
  fb1 : Inport
  fb2 : Inport  Port=2
  fb3 : Inport  Port=3
  fb4 : Inport  Port=4
  fb5 : Inport  Port=5
  fb6 : Inport  Port=6
  input : Inport  Port=7
  s1 : Inport  Port=8
  s2 : Inport  Port=9
  s3 : Inport  Port=10
  s4 : Inport  Port=11
  s5 : Inport  Port=12
  s6 : Inport  Port=13
  (I-beta*K)V_dot_est : Subsystem
  Input Processor1 : Subsystem
  KDgain1 : Subsystem
  KPgain1 : Subsystem
  KX1 : Subsystem
      settings: PortSchema="{\"entries\":[{\"content\":{\"sides\":[{\"content\":{\"connectorIds\":[\"In1\",\"In2\",\"In3\",\"In4\",\"In5\",\"In6\"]},\"type\":\"ConnectorPlacement.EquallySpacedRectSide\",\"uuid\":\"24ff0189-2e26-4de2-9c90-2043606e3d63\"},{\"content\":{\"connectorIds\":[\"Out1\",\"Out2\",\"Out3\",\"Out4\",\"Out5\",\"Out6\"],\"side\":\"RIGHT\"},\"type\":\"ConnectorPlacement.EquallySpacedRectSide\",\"uuid\":\"7efe01dd-8101-429e-adc6-a10b45356e48\"},{\"content\":{\"connectorIds\":[],\"side\":\"TOP\"},\"type\":\"ConnectorPlacement.EquallySpacedRectSide\",\"uuid\":\"5c1fc1f4-b8b0-4afd-80fe-11f4d157d0fc\"},{\"content\":{\"connectorIds\":[\"In7\",\"In8\",\"In9\",\"In10\",\"In11\",\"In12\"],\"side\":\"BOTTOM\"},\"type\":\"ConnectorPlacement.EquallySpacedRectSide\",\"uuid\":\"e52c51d8-b236-4cc8-9958-a8d91e3741c4\"}]},\"type\":\"ConnectorPlacement.EquallySpacedConnector\",\"uuid\":\"3e3502e3-b8a3-4e9d-9b78-ab08dd870d4b\"}],\"packageUris\":[\"http://schema.mathworks.com/mf0/Connector/R2020b\"],\"version\":\"1.0\"}"
  KX_dot2 : Subsystem
      settings: PortSchema="{\"entries\":[{\"content\":{\"sides\":[{\"content\":{\"connectorIds\":[\"In1\",\"In2\",\"In3\",\"In4\",\"In5\",\"In6\"]},\"type\":\"ConnectorPlacement.EquallySpacedRectSide\",\"uuid\":\"24ff0189-2e26-4de2-9c90-2043606e3d63\"},{\"content\":{\"connectorIds\":[\"Out1\",\"Out2\",\"Out3\",\"Out4\",\"Out5\",\"Out6\"],\"side\":\"RIGHT\"},\"type\":\"ConnectorPlacement.EquallySpacedRectSide\",\"uuid\":\"7efe01dd-8101-429e-adc6-a10b45356e48\"},{\"content\":{\"connectorIds\":[],\"side\":\"TOP\"},\"type\":\"ConnectorPlacement.EquallySpacedRectSide\",\"uuid\":\"5c1fc1f4-b8b0-4afd-80fe-11f4d157d0fc\"},{\"content\":{\"connectorIds\":[\"In7\",\"In8\",\"In9\",\"In10\",\"In11\",\"In12\"],\"side\":\"BOTTOM\"},\"type\":\"ConnectorPlacement.EquallySpacedRectSide\",\"uuid\":\"bae418dc-ca78-4370-85bb-31cb43009c14\"}]},\"type\":\"ConnectorPlacement.EquallySpacedConnector\",\"uuid\":\"3e3502e3-b8a3-4e9d-9b78-ab08dd870d4b\"}],\"packageUris\":[\"http://schema.mathworks.com/mf0/Connector/R2020b\"],\"version\":\"1.0\"}"
  Subsystem1 : Subsystem
  Sum{10..12,20..22} (6 alike) : Sum  Inputs=+--
  Sum13 : Sum  Inputs=++|
  Out1 : Outport
  Out2 : Outport  Port=2
  Out3 : Outport  Port=3
  Out4 : Outport  Port=4
  Out5 : Outport  Port=5
  Out6 : Outport  Port=6
  wires:
  KX_dot2/5(Output4) -> KDgain1/5(Output4)
  fb4/1 -> KX1/4(Input3), KX_dot2/4(Input3), (I-beta*K)V_dot_est/4(pos4)
  fb2/1 -> KX1/2(Input1), KX_dot2/2(Input1), (I-beta*K)V_dot_est/2(pos2)
  KDgain1/6(u5) -> Subsystem1/6(u5)
  fb3/1 -> KX1/3(Input2), KX_dot2/3(Input2), (I-beta*K)V_dot_est/3(pos3)
  KPgain1/4(Out4) -> Sum10/2
  Sum10/1 -> Out4/1
  KPgain1/2(Out2) -> Sum21/2
  KX1/6(Output5) -> KPgain1/6(Output5)
  KX1/2(Output1) -> KPgain1/2(Output1)
  KPgain1/6(Out6) -> Sum12/2
  KX1/4(Output3) -> KPgain1/4(Output3)
  KX1/3(Output2) -> KPgain1/3(Output2)
  s6/1 -> KX_dot2/12(sense6), (I-beta*K)V_dot_est/12(pos6sense), KX1/12(sense6)
  KDgain1/4(u3) -> Subsystem1/4(u3)
  fb5/1 -> KX1/5(Input4), KX_dot2/5(Input4), (I-beta*K)V_dot_est/5(pos5)
  Sum22/1 -> Out3/1
  Sum12/1 -> Out6/1
  KPgain1/3(Out3) -> Sum22/2
  KDgain1/5(u4) -> Subsystem1/5(u4)
  KDgain1/2(u1) -> Subsystem1/2(u1)
  s3/1 -> KX_dot2/9(sense3), (I-beta*K)V_dot_est/9(pos3sense), KX1/9(sense3)
  Sum20/1 -> Sum13/2
  KDgain1/3(u2) -> Subsystem1/3(u2)
  KX_dot2/4(Output3) -> KDgain1/4(Output3)
  fb1/1 -> KX1/1(Input), KX_dot2/1(Input), (I-beta*K)V_dot_est/1(pos1)
  KX_dot2/6(Output5) -> KDgain1/6(Output5)
  s1/1 -> KX_dot2/7(sense1), (I-beta*K)V_dot_est/7(pos1sense), KX1/7(sense1)
  s5/1 -> KX_dot2/11(sense5), (I-beta*K)V_dot_est/11(pos5sense), KX1/11(sense5)
  KX_dot2/2(Output1) -> KDgain1/2(Output1)
  Sum21/1 -> Out2/1
  KPgain1/5(Out5) -> Sum11/2
  fb6/1 -> KX1/6(Input5), (I-beta*K)V_dot_est/6(pos6), KX_dot2/6(Input5)
  (I-beta*K)V_dot_est/3(Output2) -> Sum22/1
  s4/1 -> KX_dot2/10(sense4), (I-beta*K)V_dot_est/10(pos4sense), KX1/10(sense4)
  KX1/5(Output4) -> KPgain1/5(Output4)
  KDgain1/1(u) -> Subsystem1/1(u)
  KX1/1(Output) -> KPgain1/1(Output)
  (I-beta*K)V_dot_est/2(Output1) -> Sum21/1
  KX_dot2/3(Output2) -> KDgain1/3(Output2)
  Sum11/1 -> Out5/1
  (I-beta*K)V_dot_est/4(Output3) -> Sum10/1
  KX_dot2/1(Output) -> KDgain1/1(Output)
  (I-beta*K)V_dot_est/5(Output4) -> Sum11/1
  (I-beta*K)V_dot_est/6(Output5) -> Sum12/1
  KPgain1/1(Out1) -> Sum20/2
  s2/1 -> KX_dot2/8(sense2), (I-beta*K)V_dot_est/8(pos2sense), KX1/8(sense2)
  Sum13/1 -> Out1/1
  Input Processor1/1(Out1) -> Sum13/1
  Subsystem1/1(Out7) -> Sum20/3
  Subsystem1/2(Out8) -> Sum21/3
  Subsystem1/3(Out9) -> Sum22/3
  Subsystem1/4(Out10) -> Sum10/3
  Subsystem1/5(Out11) -> Sum11/3
  Subsystem1/6(Out12) -> Sum12/3
  input/1 -> Input Processor1/1(Input)
  (I-beta*K)V_dot_est/1(Output) -> Sum20/1

== system DSR_delay_beta_test/Max Deflection1 ==
  In1 : Inport
  In2 : Inport  Port=2
  In3 : Inport  Port=3
  In4 : Inport  Port=4
  In5 : Inport  Port=5
  In6 : Inport  Port=6
  Abs{,1..5} (6 alike) : Abs
  Average : Subsystem
  Max : MinMax  Function=max  Inputs=6
  MinMax Running Resettable : simulink/Math Operations/MinMax Running Resettable  Function=max  vinit=0.0
  Scope3 : Scope  NumInputPorts=7
  Sum{10..13,20..21} (6 alike) : Sum  Inputs=-+|
  Zero : Constant  Value=0  OutDataTypeStr=Inherit: Inherit via back propagation
  y : Outport
  wires:
  In3/1 -> Average/3(In3), Sum12/2
  Average/1(Out1) -> Sum11/1, Sum21/1, Sum20/1, Sum13/1, Sum12/1, Sum10/1
  In1/1 -> Sum10/2, Average/1(In1)
  Max/1 -> Scope3/1, MinMax Running Resettable/1
  Abs/1 -> Max/1, Scope3/2
  Abs2/1 -> Max/3, Scope3/4
  Sum11/1 -> Abs1/1
  In2/1 -> Average/2(In2), Sum11/2
  Abs4/1 -> Scope3/6, Max/5
  Sum13/1 -> Abs3/1
  Zero/1 -> MinMax Running Resettable/2
  Sum12/1 -> Abs2/1
  Sum10/1 -> Abs/1
  In6/1 -> Sum21/2, Average/6(In6)
  In4/1 -> Average/4(In4), Sum13/2
  Abs5/1 -> Scope3/7, Max/6
  Sum21/1 -> Abs5/1
  Sum20/1 -> Abs4/1
  MinMax Running Resettable/1 -> y/1
  In5/1 -> Sum20/2, Average/5(In5)
  Abs3/1 -> Max/4, Scope3/5
  Abs1/1 -> Max/2, Scope3/3

== system DSR_delay_beta_test/Max Deflection2 ==
  In1 : Inport
  In2 : Inport  Port=2
  In3 : Inport  Port=3
  In4 : Inport  Port=4
  In5 : Inport  Port=5
  In6 : Inport  Port=6
  Abs{,1..5} (6 alike) : Abs
  Average : Subsystem
  Max : MinMax  Function=max  Inputs=6
  MinMax Running Resettable : simulink/Math Operations/MinMax Running Resettable  Function=max  vinit=0.0
  Scope3 : Scope  NumInputPorts=7
  Sum{10..13,20..21} (6 alike) : Sum  Inputs=-+|
  Zero : Constant  Value=0  OutDataTypeStr=Inherit: Inherit via back propagation
  y : Outport
  wires:
  In3/1 -> Average/3(In3), Sum12/2
  Average/1(Out1) -> Sum11/1, Sum21/1, Sum20/1, Sum13/1, Sum12/1, Sum10/1
  In1/1 -> Sum10/2, Average/1(In1)
  Max/1 -> Scope3/1, MinMax Running Resettable/1
  Abs/1 -> Max/1, Scope3/2
  Abs2/1 -> Max/3, Scope3/4
  Sum11/1 -> Abs1/1
  In2/1 -> Average/2(In2), Sum11/2
  Abs4/1 -> Scope3/6, Max/5
  Sum13/1 -> Abs3/1
  Zero/1 -> MinMax Running Resettable/2
  Sum12/1 -> Abs2/1
  Sum10/1 -> Abs/1
  In6/1 -> Sum21/2, Average/6(In6)
  In4/1 -> Average/4(In4), Sum13/2
  Abs5/1 -> Scope3/7, Max/6
  Sum21/1 -> Abs5/1
  Sum20/1 -> Abs4/1
  MinMax Running Resettable/1 -> y/1
  In5/1 -> Sum20/2, Average/5(In5)
  Abs3/1 -> Max/4, Scope3/5
  Abs1/1 -> Max/2, Scope3/3

== system DSR_delay_beta_test/Max Deflection3 ==
  In1 : Inport
  In2 : Inport  Port=2
  In3 : Inport  Port=3
  In4 : Inport  Port=4
  In5 : Inport  Port=5
  In6 : Inport  Port=6
  Abs{,1..5} (6 alike) : Abs
  Average : Subsystem
  Max : MinMax  Function=max  Inputs=6
  MinMax Running Resettable : simulink/Math Operations/MinMax Running Resettable  Function=max  vinit=0.0
  Scope3 : Scope  NumInputPorts=7
  Sum{10..13,20..21} (6 alike) : Sum  Inputs=-+|
  Zero : Constant  Value=0  OutDataTypeStr=Inherit: Inherit via back propagation
  y : Outport
  wires:
  In3/1 -> Average/3(In3), Sum12/2
  Average/1(Out1) -> Sum11/1, Sum21/1, Sum20/1, Sum13/1, Sum12/1, Sum10/1
  In1/1 -> Sum10/2, Average/1(In1)
  Max/1 -> Scope3/1, MinMax Running Resettable/1
  Abs/1 -> Max/1, Scope3/2
  Abs2/1 -> Max/3, Scope3/4
  Sum11/1 -> Abs1/1
  In2/1 -> Average/2(In2), Sum11/2
  Abs4/1 -> Scope3/6, Max/5
  Sum13/1 -> Abs3/1
  Zero/1 -> MinMax Running Resettable/2
  Sum12/1 -> Abs2/1
  Sum10/1 -> Abs/1
  In6/1 -> Sum21/2, Average/6(In6)
  In4/1 -> Average/4(In4), Sum13/2
  Abs5/1 -> Scope3/7, Max/6
  Sum21/1 -> Abs5/1
  Sum20/1 -> Abs4/1
  MinMax Running Resettable/1 -> y/1
  In5/1 -> Sum20/2, Average/5(In5)
  Abs3/1 -> Max/4, Scope3/5
  Abs1/1 -> Max/2, Scope3/3

== system DSR_delay_beta_test/StateDerivative1 ==
  Input : Inport
  Input1 : Inport  Port=2
  Input2 : Inport  Port=3
  Input3 : Inport  Port=4
  Input4 : Inport  Port=5
  Input5 : Inport  Port=6
  Derivative{,1..5} (6 alike) : Derivative
  Varying Lowpass Filter{,1..5} (6 alike) : cstblocks/Linear Parameter Varying/Varying Lowpass Filter  N=1
  Zero : Constant  Value=omegader  OutDataTypeStr=Inherit: Inherit via back propagation
  Out1 : Outport
  Out2 : Outport  Port=2
  Out3 : Outport  Port=3
  Out4 : Outport  Port=4
  Out5 : Outport  Port=5
  Out6 : Outport  Port=6
  wires:
  Input2/1 -> Derivative2/1
  Input/1 -> Derivative/1
  Input1/1 -> Derivative1/1
  Input4/1 -> Derivative4/1
  Input3/1 -> Derivative3/1
  Input5/1 -> Derivative5/1
  Derivative/1 -> Varying Lowpass Filter/1
  Derivative1/1 -> Varying Lowpass Filter1/1
  Derivative2/1 -> Varying Lowpass Filter2/1
  Derivative3/1 -> Varying Lowpass Filter3/1
  Derivative4/1 -> Varying Lowpass Filter4/1
  Derivative5/1 -> Varying Lowpass Filter5/1
  Varying Lowpass Filter/1 -> Out1/1
  Varying Lowpass Filter1/1 -> Out2/1
  Varying Lowpass Filter2/1 -> Out3/1
  Varying Lowpass Filter3/1 -> Out4/1
  Varying Lowpass Filter4/1 -> Out5/1
  Varying Lowpass Filter5/1 -> Out6/1
  Zero/1 -> Varying Lowpass Filter3/2, Varying Lowpass Filter/2, Varying Lowpass Filter1/2, Varying Lowpass Filter2/2, Varying Lowpass Filter4/2, Varying Lowpass Filter5/2

== system DSR_delay_beta_test/StateDerivative2 ==
  Input : Inport
  Input1 : Inport  Port=2
  Input2 : Inport  Port=3
  Input3 : Inport  Port=4
  Input4 : Inport  Port=5
  Input5 : Inport  Port=6
  Derivative{,1..5} (6 alike) : Derivative
  Varying Lowpass Filter{,1..5} (6 alike) : cstblocks/Linear Parameter Varying/Varying Lowpass Filter  N=1
  Zero : Constant  Value=omegader  OutDataTypeStr=Inherit: Inherit via back propagation
  Out1 : Outport
  Out2 : Outport  Port=2
  Out3 : Outport  Port=3
  Out4 : Outport  Port=4
  Out5 : Outport  Port=5
  Out6 : Outport  Port=6
  wires:
  Input2/1 -> Derivative2/1
  Input/1 -> Derivative/1
  Input1/1 -> Derivative1/1
  Input4/1 -> Derivative4/1
  Input3/1 -> Derivative3/1
  Input5/1 -> Derivative5/1
  Derivative/1 -> Varying Lowpass Filter/1
  Derivative1/1 -> Varying Lowpass Filter1/1
  Derivative2/1 -> Varying Lowpass Filter2/1
  Derivative3/1 -> Varying Lowpass Filter3/1
  Derivative4/1 -> Varying Lowpass Filter4/1
  Derivative5/1 -> Varying Lowpass Filter5/1
  Varying Lowpass Filter/1 -> Out1/1
  Varying Lowpass Filter1/1 -> Out2/1
  Varying Lowpass Filter2/1 -> Out3/1
  Varying Lowpass Filter3/1 -> Out4/1
  Varying Lowpass Filter4/1 -> Out5/1
  Varying Lowpass Filter5/1 -> Out6/1
  Zero/1 -> Varying Lowpass Filter3/2, Varying Lowpass Filter/2, Varying Lowpass Filter1/2, Varying Lowpass Filter2/2, Varying Lowpass Filter4/2, Varying Lowpass Filter5/2

== system DSR_delay_beta_test/StateDerivative3 ==
  Input : Inport
  Input1 : Inport  Port=2
  Input2 : Inport  Port=3
  Input3 : Inport  Port=4
  Input4 : Inport  Port=5
  Input5 : Inport  Port=6
  Derivative{,1..5} (6 alike) : Derivative
  Varying Lowpass Filter{,1..5} (6 alike) : cstblocks/Linear Parameter Varying/Varying Lowpass Filter  N=1
  Zero : Constant  Value=omegader  OutDataTypeStr=Inherit: Inherit via back propagation
  Out1 : Outport
  Out2 : Outport  Port=2
  Out3 : Outport  Port=3
  Out4 : Outport  Port=4
  Out5 : Outport  Port=5
  Out6 : Outport  Port=6
  wires:
  Input2/1 -> Derivative2/1
  Input/1 -> Derivative/1
  Input1/1 -> Derivative1/1
  Input4/1 -> Derivative4/1
  Input3/1 -> Derivative3/1
  Input5/1 -> Derivative5/1
  Derivative/1 -> Varying Lowpass Filter/1
  Derivative1/1 -> Varying Lowpass Filter1/1
  Derivative2/1 -> Varying Lowpass Filter2/1
  Derivative3/1 -> Varying Lowpass Filter3/1
  Derivative4/1 -> Varying Lowpass Filter4/1
  Derivative5/1 -> Varying Lowpass Filter5/1
  Varying Lowpass Filter/1 -> Out1/1
  Varying Lowpass Filter1/1 -> Out2/1
  Varying Lowpass Filter2/1 -> Out3/1
  Varying Lowpass Filter3/1 -> Out4/1
  Varying Lowpass Filter4/1 -> Out5/1
  Varying Lowpass Filter5/1 -> Out6/1
  Zero/1 -> Varying Lowpass Filter3/2, Varying Lowpass Filter/2, Varying Lowpass Filter1/2, Varying Lowpass Filter2/2, Varying Lowpass Filter4/2, Varying Lowpass Filter5/2

== system DSR_delay_beta_test/Subsystem1 ==
  In1 : Inport
  In2 : Inport  Port=2
  In3 : Inport  Port=3
  In4 : Inport  Port=4
  In5 : Inport  Port=5
  In6 : Inport  Port=6
  Transfer Fcn{,1..5} (6 alike) : TransferFcn  Numerator=[a]  Denominator=[1 a 0]
  O1 : Outport
  O2 : Outport  Port=2
  O3 : Outport  Port=3
  O4 : Outport  Port=4
  O5 : Outport  Port=5
  O6 : Outport  Port=6
  wires:
  Transfer Fcn1/1 -> O2/1
  In1/1 -> Transfer Fcn/1
  Transfer Fcn/1 -> O1/1
  In4/1 -> Transfer Fcn3/1
  Transfer Fcn3/1 -> O4/1
  In3/1 -> Transfer Fcn2/1
  In2/1 -> Transfer Fcn1/1
  Transfer Fcn2/1 -> O3/1
  Transfer Fcn5/1 -> O6/1
  In6/1 -> Transfer Fcn5/1
  In5/1 -> Transfer Fcn4/1
  Transfer Fcn4/1 -> O5/1

== system DSR_delay_beta_test/Subsystem2 ==
  In1 : Inport
  In2 : Inport  Port=2
  In3 : Inport  Port=3
  In4 : Inport  Port=4
  In5 : Inport  Port=5
  In6 : Inport  Port=6
  Transfer Fcn{,1..5} (6 alike) : TransferFcn  Numerator=[a]  Denominator=[1 a 0]
  O1 : Outport
  O2 : Outport  Port=2
  O3 : Outport  Port=3
  O4 : Outport  Port=4
  O5 : Outport  Port=5
  O6 : Outport  Port=6
  wires:
  Transfer Fcn1/1 -> O2/1
  In1/1 -> Transfer Fcn/1
  Transfer Fcn/1 -> O1/1
  In4/1 -> Transfer Fcn3/1
  Transfer Fcn3/1 -> O4/1
  In3/1 -> Transfer Fcn2/1
  In2/1 -> Transfer Fcn1/1
  Transfer Fcn2/1 -> O3/1
  Transfer Fcn5/1 -> O6/1
  In6/1 -> Transfer Fcn5/1
  In5/1 -> Transfer Fcn4/1
  Transfer Fcn4/1 -> O5/1

== system DSR_delay_beta_test/Subsystem3 ==
  In1 : Inport
  In2 : Inport  Port=2
  In3 : Inport  Port=3
  In4 : Inport  Port=4
  In5 : Inport  Port=5
  In6 : Inport  Port=6
  Transfer Fcn{,1..5} (6 alike) : TransferFcn  Numerator=[a]  Denominator=[1 a 0]
  O1 : Outport
  O2 : Outport  Port=2
  O3 : Outport  Port=3
  O4 : Outport  Port=4
  O5 : Outport  Port=5
  O6 : Outport  Port=6
  wires:
  Transfer Fcn1/1 -> O2/1
  In1/1 -> Transfer Fcn/1
  Transfer Fcn/1 -> O1/1
  In4/1 -> Transfer Fcn3/1
  Transfer Fcn3/1 -> O4/1
  In3/1 -> Transfer Fcn2/1
  In2/1 -> Transfer Fcn1/1
  Transfer Fcn2/1 -> O3/1
  Transfer Fcn5/1 -> O6/1
  In6/1 -> Transfer Fcn5/1
  In5/1 -> Transfer Fcn4/1
  Transfer Fcn4/1 -> O5/1

== system DSR_delay_beta_test/gain 1//a1 ==
  In1 : Inport
  In2 : Inport  Port=2
  In3 : Inport  Port=3
  In4 : Inport  Port=4
  In5 : Inport  Port=5
  In6 : Inport  Port=6
  1/a{,1..5} (6 alike) : Gain  Gain=1/a
  Out1 : Outport
  Out2 : Outport  Port=2
  Out3 : Outport  Port=3
  Out4 : Outport  Port=4
  Out5 : Outport  Port=5
  Out6 : Outport  Port=6
  wires:
  1/a2/1 -> Out3/1
  In1/1 -> 1/a/1
  In4/1 -> 1/a3/1
  1/a5/1 -> Out6/1
  In2/1 -> 1/a1/1
  1/a4/1 -> Out5/1
  1/a/1 -> Out1/1
  In6/1 -> 1/a5/1
  1/a3/1 -> Out4/1
  In5/1 -> 1/a4/1
  In3/1 -> 1/a2/1
  1/a1/1 -> Out2/1

== system DSR_delay_beta_test/gain 1//a2 ==
  In1 : Inport
  In2 : Inport  Port=2
  In3 : Inport  Port=3
  In4 : Inport  Port=4
  In5 : Inport  Port=5
  In6 : Inport  Port=6
  1/a{,1..5} (6 alike) : Gain  Gain=1/a
  Out1 : Outport
  Out2 : Outport  Port=2
  Out3 : Outport  Port=3
  Out4 : Outport  Port=4
  Out5 : Outport  Port=5
  Out6 : Outport  Port=6
  wires:
  1/a2/1 -> Out3/1
  In1/1 -> 1/a/1
  In4/1 -> 1/a3/1
  1/a5/1 -> Out6/1
  In2/1 -> 1/a1/1
  1/a4/1 -> Out5/1
  1/a/1 -> Out1/1
  In6/1 -> 1/a5/1
  1/a3/1 -> Out4/1
  In5/1 -> 1/a4/1
  In3/1 -> 1/a2/1
  1/a1/1 -> Out2/1

== system DSR_delay_beta_test/gain 1//a3 ==
  In1 : Inport
  In2 : Inport  Port=2
  In3 : Inport  Port=3
  In4 : Inport  Port=4
  In5 : Inport  Port=5
  In6 : Inport  Port=6
  1/a{,1..5} (6 alike) : Gain  Gain=1/a
  Out1 : Outport
  Out2 : Outport  Port=2
  Out3 : Outport  Port=3
  Out4 : Outport  Port=4
  Out5 : Outport  Port=5
  Out6 : Outport  Port=6
  wires:
  1/a2/1 -> Out3/1
  In1/1 -> 1/a/1
  In4/1 -> 1/a3/1
  1/a5/1 -> Out6/1
  In2/1 -> 1/a1/1
  1/a4/1 -> Out5/1
  1/a/1 -> Out1/1
  In6/1 -> 1/a5/1
  1/a3/1 -> Out4/1
  In5/1 -> 1/a4/1
  In3/1 -> 1/a2/1
  1/a1/1 -> Out2/1

== system DSR_delay_beta_test/CDOB_Subsys1/ND ==
  XRes : Inport
  Acc. : Inport  Port=2
  CDOB1 : Subsystem
  TimeDelayComp : Subsystem
  FeedBack : Outport
  wires:
  CDOB1/1(Dobsv) -> TimeDelayComp/2(Dobsv)
  Acc./1 -> CDOB1/2(Acc.)
  TimeDelayComp/1(FeedBack) -> FeedBack/1
  XRes/1 -> TimeDelayComp/1(SysOut), CDOB1/1(XRes)

== system DSR_delay_beta_test/CDOB_Subsys1/ND1 ==
  XRes : Inport
  Acc. : Inport  Port=2
  CDOB1 : Subsystem
  TimeDelayComp : Subsystem
  FeedBack : Outport
  wires:
  CDOB1/1(Dobsv) -> TimeDelayComp/2(Dobsv)
  Acc./1 -> CDOB1/2(Acc.)
  TimeDelayComp/1(FeedBack) -> FeedBack/1
  XRes/1 -> TimeDelayComp/1(SysOut), CDOB1/1(XRes)

== system DSR_delay_beta_test/CDOB_Subsys1/ND2 ==
  XRes : Inport
  Acc. : Inport  Port=2
  CDOB1 : Subsystem
  TimeDelayComp : Subsystem
  FeedBack : Outport
  wires:
  CDOB1/1(Dobsv) -> TimeDelayComp/2(Dobsv)
  Acc./1 -> CDOB1/2(Acc.)
  TimeDelayComp/1(FeedBack) -> FeedBack/1
  XRes/1 -> TimeDelayComp/1(SysOut), CDOB1/1(XRes)

== system DSR_delay_beta_test/CDOB_Subsys1/ND3 ==
  XRes : Inport
  Acc. : Inport  Port=2
  CDOB1 : Subsystem
  TimeDelayComp : Subsystem
  FeedBack : Outport
  wires:
  CDOB1/1(Dobsv) -> TimeDelayComp/2(Dobsv)
  Acc./1 -> CDOB1/2(Acc.)
  TimeDelayComp/1(FeedBack) -> FeedBack/1
  XRes/1 -> TimeDelayComp/1(SysOut), CDOB1/1(XRes)

== system DSR_delay_beta_test/CDOB_Subsys1/ND4 ==
  XRes : Inport
  Acc. : Inport  Port=2
  CDOB1 : Subsystem
  TimeDelayComp : Subsystem
  FeedBack : Outport
  wires:
  CDOB1/1(Dobsv) -> TimeDelayComp/2(Dobsv)
  Acc./1 -> CDOB1/2(Acc.)
  TimeDelayComp/1(FeedBack) -> FeedBack/1
  XRes/1 -> TimeDelayComp/1(SysOut), CDOB1/1(XRes)

== system DSR_delay_beta_test/CDOB_Subsys1/ND5 ==
  XRes : Inport
  Acc. : Inport  Port=2
  CDOB1 : Subsystem
  TimeDelayComp : Subsystem
  FeedBack : Outport
  wires:
  CDOB1/1(Dobsv) -> TimeDelayComp/2(Dobsv)
  Acc./1 -> CDOB1/2(Acc.)
  TimeDelayComp/1(FeedBack) -> FeedBack/1
  XRes/1 -> TimeDelayComp/1(SysOut), CDOB1/1(XRes)

== system DSR_delay_beta_test/CDOB_Subsys2/ND ==
  XRes : Inport
  Acc. : Inport  Port=2
  CDOB1 : Subsystem
  TimeDelayComp : Subsystem
  FeedBack : Outport
  wires:
  CDOB1/1(Dobsv) -> TimeDelayComp/2(Dobsv)
  Acc./1 -> CDOB1/2(Acc.)
  TimeDelayComp/1(FeedBack) -> FeedBack/1
  XRes/1 -> TimeDelayComp/1(SysOut), CDOB1/1(XRes)

== system DSR_delay_beta_test/CDOB_Subsys2/ND1 ==
  XRes : Inport
  Acc. : Inport  Port=2
  CDOB1 : Subsystem
  TimeDelayComp : Subsystem
  FeedBack : Outport
  wires:
  CDOB1/1(Dobsv) -> TimeDelayComp/2(Dobsv)
  Acc./1 -> CDOB1/2(Acc.)
  TimeDelayComp/1(FeedBack) -> FeedBack/1
  XRes/1 -> TimeDelayComp/1(SysOut), CDOB1/1(XRes)

== system DSR_delay_beta_test/CDOB_Subsys2/ND2 ==
  XRes : Inport
  Acc. : Inport  Port=2
  CDOB1 : Subsystem
  TimeDelayComp : Subsystem
  FeedBack : Outport
  wires:
  CDOB1/1(Dobsv) -> TimeDelayComp/2(Dobsv)
  Acc./1 -> CDOB1/2(Acc.)
  TimeDelayComp/1(FeedBack) -> FeedBack/1
  XRes/1 -> TimeDelayComp/1(SysOut), CDOB1/1(XRes)

== system DSR_delay_beta_test/CDOB_Subsys2/ND3 ==
  XRes : Inport
  Acc. : Inport  Port=2
  CDOB1 : Subsystem
  TimeDelayComp : Subsystem
  FeedBack : Outport
  wires:
  CDOB1/1(Dobsv) -> TimeDelayComp/2(Dobsv)
  Acc./1 -> CDOB1/2(Acc.)
  TimeDelayComp/1(FeedBack) -> FeedBack/1
  XRes/1 -> TimeDelayComp/1(SysOut), CDOB1/1(XRes)

== system DSR_delay_beta_test/CDOB_Subsys2/ND4 ==
  XRes : Inport
  Acc. : Inport  Port=2
  CDOB1 : Subsystem
  TimeDelayComp : Subsystem
  FeedBack : Outport
  wires:
  CDOB1/1(Dobsv) -> TimeDelayComp/2(Dobsv)
  Acc./1 -> CDOB1/2(Acc.)
  TimeDelayComp/1(FeedBack) -> FeedBack/1
  XRes/1 -> TimeDelayComp/1(SysOut), CDOB1/1(XRes)

== system DSR_delay_beta_test/CDOB_Subsys2/ND5 ==
  XRes : Inport
  Acc. : Inport  Port=2
  CDOB1 : Subsystem
  TimeDelayComp : Subsystem
  FeedBack : Outport
  wires:
  CDOB1/1(Dobsv) -> TimeDelayComp/2(Dobsv)
  Acc./1 -> CDOB1/2(Acc.)
  TimeDelayComp/1(FeedBack) -> FeedBack/1
  XRes/1 -> TimeDelayComp/1(SysOut), CDOB1/1(XRes)

== system DSR_delay_beta_test/CDOB_Subsys4/ND ==
  XRes : Inport
  Acc. : Inport  Port=2
  CDOB1 : Subsystem
  TimeDelayComp : Subsystem
  FeedBack : Outport
  wires:
  CDOB1/1(Dobsv) -> TimeDelayComp/2(Dobsv)
  Acc./1 -> CDOB1/2(Acc.)
  TimeDelayComp/1(FeedBack) -> FeedBack/1
  XRes/1 -> TimeDelayComp/1(SysOut), CDOB1/1(XRes)

== system DSR_delay_beta_test/CDOB_Subsys4/ND1 ==
  XRes : Inport
  Acc. : Inport  Port=2
  CDOB1 : Subsystem
  TimeDelayComp : Subsystem
  FeedBack : Outport
  wires:
  CDOB1/1(Dobsv) -> TimeDelayComp/2(Dobsv)
  Acc./1 -> CDOB1/2(Acc.)
  TimeDelayComp/1(FeedBack) -> FeedBack/1
  XRes/1 -> TimeDelayComp/1(SysOut), CDOB1/1(XRes)

== system DSR_delay_beta_test/CDOB_Subsys4/ND2 ==
  XRes : Inport
  Acc. : Inport  Port=2
  CDOB1 : Subsystem
  TimeDelayComp : Subsystem
  FeedBack : Outport
  wires:
  CDOB1/1(Dobsv) -> TimeDelayComp/2(Dobsv)
  Acc./1 -> CDOB1/2(Acc.)
  TimeDelayComp/1(FeedBack) -> FeedBack/1
  XRes/1 -> TimeDelayComp/1(SysOut), CDOB1/1(XRes)

== system DSR_delay_beta_test/CDOB_Subsys4/ND3 ==
  XRes : Inport
  Acc. : Inport  Port=2
  CDOB1 : Subsystem
  TimeDelayComp : Subsystem
  FeedBack : Outport
  wires:
  CDOB1/1(Dobsv) -> TimeDelayComp/2(Dobsv)
  Acc./1 -> CDOB1/2(Acc.)
  TimeDelayComp/1(FeedBack) -> FeedBack/1
  XRes/1 -> TimeDelayComp/1(SysOut), CDOB1/1(XRes)

== system DSR_delay_beta_test/CDOB_Subsys4/ND4 ==
  XRes : Inport
  Acc. : Inport  Port=2
  CDOB1 : Subsystem
  TimeDelayComp : Subsystem
  FeedBack : Outport
  wires:
  CDOB1/1(Dobsv) -> TimeDelayComp/2(Dobsv)
  Acc./1 -> CDOB1/2(Acc.)
  TimeDelayComp/1(FeedBack) -> FeedBack/1
  XRes/1 -> TimeDelayComp/1(SysOut), CDOB1/1(XRes)
